simulink model "lab6_1_sim"  (R2018a)
settings: Solver=VariableStepAuto  StartTime=0.0  StopTime=10.0  RelTol=1e-3
values from neighbouring files (symbols this model uses):
  b = 1    [lab6_1.m]
  ksi = 1    [lab6_1.m]
  w = 1    [lab6_1.m]
settings Model: Creator=john  LastModifiedBy=john

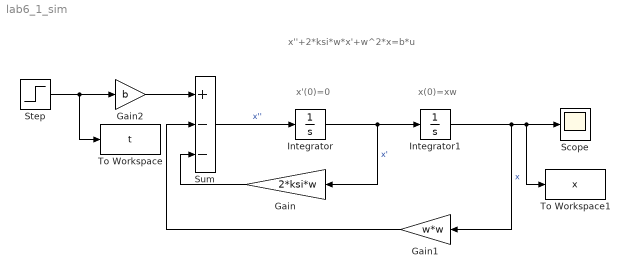
== system lab6_1_sim ==
  note: x(0)=xw
  note: x'(0)=0
  note: x''+2*ksi*w*x'+w^2*x=b*u
  Gain : Gain  Gain=2*ksi*w
  Gain1 : Gain  Gain=w*w
  Gain2 : Gain  Gain=b
  Integrator : Integrator
  Integrator1 : Integrator  InitialCondition=b/(w*w)
  Scope : Scope
  Step : Step  Before=1  SampleTime=0
  Sum : Sum  Inputs=+--
  To Workspace : ToWorkspace  VariableName=t  SaveFormat=Timeseries  SampleTime=-1
  To Workspace1 : ToWorkspace  VariableName=x  SampleTime=-1
  wires:
  Integrator/1 -> Gain/1, Integrator1/1  "x'"
  Integrator1/1 -> Gain1/1, To Workspace1/1, Scope/1  "x"
  Sum/1 -> Integrator/1  "x''"
  Gain/1 -> Sum/3
  Gain1/1 -> Sum/2
  Step/1 -> To Workspace/1, Gain2/1
  Gain2/1 -> Sum/1
